simulink model "simulink1"  (R2017b)
settings: Solver=VariableStepAuto  StartTime=0.0  StopTime=20  RelTol=1e-3
values from neighbouring files (symbols this model uses):
  P = [1 -p1 -p2]    [uloha1.m]
  P1 = [1 p1 p2]    [uloha1.m]
  Q = [q0 q1]    [uloha1.m]
settings Model: Creator=jan.sedivy  LastModifiedBy=jan.sedivy

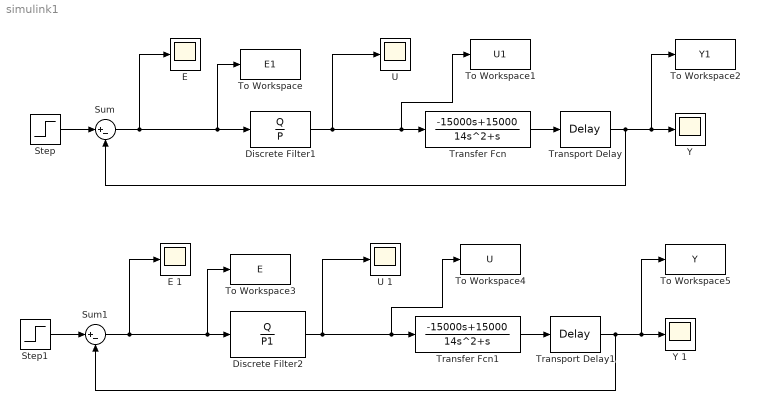
== system simulink1 ==
  Discrete Filter1 : DiscreteFilter  Numerator=Q  Denominator=P  SampleTime=4
  Discrete Filter2 : DiscreteFilter  Numerator=Q  Denominator=P1  SampleTime=1
  "E " : Scope
  E 1 : Scope
  Step : Step  Time=0  SampleTime=0
  Step1 : Step  Time=0  SampleTime=0
  Sum : Sum  Inputs=|+-
  Sum1 : Sum  Inputs=|+-
  To Workspace : ToWorkspace  VariableName=E1  SaveFormat=Timeseries  SampleTime=-1
  To Workspace1 : ToWorkspace  VariableName=U1  SaveFormat=Timeseries  SampleTime=-1
  To Workspace2 : ToWorkspace  VariableName=Y1  SaveFormat=Timeseries  SampleTime=-1
  To Workspace3 : ToWorkspace  VariableName=E  SaveFormat=Timeseries  SampleTime=-1
  To Workspace4 : ToWorkspace  VariableName=U  SaveFormat=Timeseries  SampleTime=-1
  To Workspace5 : ToWorkspace  VariableName=Y  SaveFormat=Timeseries  SampleTime=-1
  Transfer Fcn : TransferFcn  Numerator=[-15000 15000]  Denominator=[14 1 0]
  Transfer Fcn1 : TransferFcn  Numerator=[-15000 15000]  Denominator=[14 1 0]
  Transport Delay : TransportDelay  DelayTime=4
  Transport Delay1 : TransportDelay
  "U " : Scope
  U 1 : Scope
  "Y " : Scope
  Y 1 : Scope
  wires:
  Transport Delay1/1 -> Sum1/2, To Workspace5/1, Y 1/1
  Transport Delay/1 -> Sum/2, To Workspace2/1, "Y "/1
  Transfer Fcn1/1 -> Transport Delay1/1
  Discrete Filter2/1 -> To Workspace4/1, Transfer Fcn1/1, U 1/1
  Discrete Filter1/1 -> "U "/1, To Workspace1/1, Transfer Fcn/1
  Step1/1 -> Sum1/1
  Transfer Fcn/1 -> Transport Delay/1
  Step/1 -> Sum/1
  Sum1/1 -> To Workspace3/1, Discrete Filter2/1, E 1/1
  Sum/1 -> Discrete Filter1/1, To Workspace/1, "E "/1
